simulink model "bus_as_currentsource_charging_discharging_battery_1"  (R2023a)
settings: Solver=VariableStepAuto  StartTime=0.0  StopTime=0.01  RelTol=1e-3
libraries: spsParallelRLCBranchLib x72, spsCurrentMeasurementLib x27, spsVoltageMeasurementLib x27, spspowerguiLib x25, spsControlledVoltageSourceLib x24, spsVariableResistorLib x24, spsSeriesRLCBranchLib x6, spsMosfetLib x2, sdolib x1, spsControlledCurrentSourceLib x1, spsGroundLib x1
(part 3 of 4)

== system bus_as_currentsource_charging_discharging_battery_1/Subsystem24 ==
  Clock : Clock
  Controlled Voltage Source : spsControlledVoltageSourceLib/Controlled Voltage Source  Initialize=on  Source_Type=DC  Amplitude=0  Phase=0  Frequency=0  Measurements=None
  Current Measurement : spsCurrentMeasurementLib/Current Measurement  PhasorSimulation=off  OutputType=Complex  PSBequivalent=0
  Delay : Delay  DelayLength=1  InitialCondition=0
  Delay1 : Delay  DelayLength=1  InitialCondition=0
  From1 : From
  From3 : From
  Goto1 : Goto
  Integrator : Integrator
  MATLAB Function : MATLAB Function  TreatAsAtomicUnit=on
  MATLAB Function1 : MATLAB Function  TreatAsAtomicUnit=on
  MATLAB Function2 : MATLAB Function  TreatAsAtomicUnit=on
  Parallel RLC Branch : spsParallelRLCBranchLib/Parallel RLC Branch  LConnTagsString=a  RConnTagsString=__new0  BranchType=RC  Resistance=15.5e-3  Inductance=1e-3  SetiL0=off  InitialCurrent=0  Capacitance=1028.7  Setx0=off  InitialVoltage=0  Measurements=None
  Parallel RLC Branch1 : spsParallelRLCBranchLib/Parallel RLC Branch  LConnTagsString=a  RConnTagsString=__new0  BranchType=RC  Resistance=18.3e-3  Inductance=1e-3  SetiL0=off  InitialCurrent=0  Capacitance=5756.6  Setx0=off  InitialVoltage=0  Measurements=None
  Parallel RLC Branch2 : spsParallelRLCBranchLib/Parallel RLC Branch  LConnTagsString=a  RConnTagsString=__new0  BranchType=R  Resistance=1e9  Inductance=1e-3  SetiL0=off  InitialCurrent=0  Capacitance=5756.6  Setx0=off  InitialVoltage=0  Measurements=None
  Scope2 : Scope
  Scope3 : Scope
  Scope4 : Scope
  Variable Resistor : spsVariableResistorLib/Variable Resistor  Rabsmin=1e-3
      settings: LibrarySourceBlock=sps_lib/Passives/Variable Resistor
  Voltage Measurement1 : spsVoltageMeasurementLib/Voltage Measurement  PhasorSimulation=off  OutputType=Complex  PSBequivalent=0
  XY Graph : Record  FileSettingsInternal="{\"entries\":[{\"content\":{\"excelSettings\":{\"content\":{},\"type\":\"Streamout.ExcelSettings\"}},\"type\":\"Streamout.FileSettingStorage\",\"uuid\":\"c5b1bd46-5ad2-463b-b602-37259b8cdc8f\"}],\"packageUris\":[\"http://schema.mathworks.com/mf0/streamout_blocks/R2020a\"],\"version\":\"1.0\"}"  Layout=[1 1]  SignalsInternal="{\"entries\":[{\"content\":{\"signals\":[{\"content\":{\"blockPath\":[\"bus_as_currentsource_charging_discharging_battery_1/Subsystem24/XY Graph\"],\"dimensions\":[1],\"domain\":\"bus_as_currentsource_charging_discharging_battery_1/Subsystem24/XY Graph\",\"lineColor\":\"#64d413\",\"port\":1,\"sid\":[\"\"],\"signalID\":331,\"signalName\":\"MATLAB Function2\"},\"type\":\"RecordBlkView.Signal\",\"uuid\":\"53831fb7-9f58-4ff5-bfff-82d8b3aa7aac\"},{\"content\":{\"blockPath\":[\"bus_as_currentsource_charging_discharging_battery_1/Subsystem24/XY Graph\"],\"dimensions\":[1],\"domain\":\"bus_as_currentsource_charging_discharging_battery_1/Subsystem24/XY Graph\",\"lineColor\":\"#ff13a6\",\"port\":2,\"sid\":[\"\"],\"signalID\":335,\"signalName\":\"Voltage Measurement1\"},\"type\":\"RecordBlkView.Signal\",\"uuid\":\"f3f18b01-4fe8-49fc-91c3-b068602f11c8\"}]},\"type\":\"RecordBlkView.InputSignals\",\"uuid\":\"28f569b0-f03a-459d-a4e3-dabbf623ccbc\"}],\"packageUris\":[\"http://schema.mathworks.com/mf0/streamout_blocks/R2020a\"],\"version\":\"1.0\"}"  VisualizationBindings="{\"xyplotplugin\":{\"info\":[{\"series\":[],\"subplotID\":1}]}}"  CompatibilityTag=XY
  powergui1 : spspowerguiLib/powergui  Priority=1  SimulationMode=Discrete  SampleTime=2e-7  frequency=60  Iterations=50  frequencyindice=0  Pbase=100e6  ErrMax=1e-4  UnitsV=kV  UnitsW=MW  buscounter=0  FunctionMessages=off  echomessages=off  EnableUseOfTLC=off  CurrentSourceSwitches=off  DisableSnubberDevices=off  DisableRonSwitches=off  DisableVfSwitches=off  DisplayEquations=off  AutomaticDiscreteSolvers=off  SolverType=Tustin/Backward Euler (TBE)  Interpol=off  ExternalGateDelay=off  methode=off  Ts=100  x0status=blocks  SPID=on  SwTol=0  HookPort=off  NonlinearTolerance=1e-4  nMaxIteration=100  ContinueOnMaxIteration=off  RestoreLinks=warning  ResistiveCurrentMeasurement=off  Frange=[0:2:500]  Ylog=off  Xlog=on  ShowGrid=off  save=off  variable=ZData  structure=0  ZoomFFT=off  StartTime=0.0  cycles=1  DisplayStyle=1  fundamental=60  FreqAxis=off  MaxFrequency=1000  frequencyindicesteady=1  RmsSteady=1  display=off
  + : PMIOPort  Side=Right
  - : PMIOPort  Port=2  Side=Left
  wires:
  Current Measurement/1 -> Goto1/1
  From3/1 -> Scope3/1
  Voltage Measurement1/1 -> XY Graph/2, Scope2/1
  MATLAB Function2/1(SOC) -> Delay/1, XY Graph/1, Scope4/1
  From1/1 -> Integrator/1
  MATLAB Function/1(y) -> Controlled Voltage Source/1
  MATLAB Function1/1(y) -> Variable Resistor/1
  Integrator/1 -> MATLAB Function2/1(u), MATLAB Function/1(u)
  Clock/1 -> MATLAB Function2/2(time), MATLAB Function/2(time)
  MATLAB Function/2(SOC) -> Delay1/1, MATLAB Function1/1(SOC)
  Delay/1 -> MATLAB Function2/3(SOC1)
  Delay1/1 -> MATLAB Function/3(SOC1)
  connections:
  Variable Resistor/RConn1 -- Parallel RLC Branch/LConn1
  Parallel RLC Branch1/RConn1 -- Parallel RLC Branch2/LConn1 -- +/RConn1 -- Voltage Measurement1/LConn1
  Voltage Measurement1/LConn2 -- Parallel RLC Branch2/RConn1 -- -/RConn1 -- Current Measurement/LConn1
  Controlled Voltage Source/RConn1 -- Variable Resistor/LConn1
  Current Measurement/RConn1 -- Controlled Voltage Source/LConn1
  Parallel RLC Branch/RConn1 -- Parallel RLC Branch1/LConn1

== system bus_as_currentsource_charging_discharging_battery_1/Subsystem3 ==
  Clock : Clock
  Controlled Voltage Source : spsControlledVoltageSourceLib/Controlled Voltage Source  Initialize=on  Source_Type=DC  Amplitude=0  Phase=0  Frequency=0  Measurements=None
  Current Measurement : spsCurrentMeasurementLib/Current Measurement  PhasorSimulation=off  OutputType=Complex  PSBequivalent=0
  Delay : Delay  DelayLength=1  InitialCondition=0
  Delay1 : Delay  DelayLength=1  InitialCondition=0
  From1 : From
  From3 : From
  Goto1 : Goto
  Integrator : Integrator
  MATLAB Function : MATLAB Function  TreatAsAtomicUnit=on
  MATLAB Function1 : MATLAB Function  TreatAsAtomicUnit=on
  MATLAB Function2 : MATLAB Function  TreatAsAtomicUnit=on
  Parallel RLC Branch : spsParallelRLCBranchLib/Parallel RLC Branch  LConnTagsString=a  RConnTagsString=__new0  BranchType=RC  Resistance=15.5e-3  Inductance=1e-3  SetiL0=off  InitialCurrent=0  Capacitance=1028.7  Setx0=off  InitialVoltage=0  Measurements=None
  Parallel RLC Branch1 : spsParallelRLCBranchLib/Parallel RLC Branch  LConnTagsString=a  RConnTagsString=__new0  BranchType=RC  Resistance=18.3e-3  Inductance=1e-3  SetiL0=off  InitialCurrent=0  Capacitance=5756.6  Setx0=off  InitialVoltage=0  Measurements=None
  Parallel RLC Branch2 : spsParallelRLCBranchLib/Parallel RLC Branch  LConnTagsString=a  RConnTagsString=__new0  BranchType=R  Resistance=1e9  Inductance=1e-3  SetiL0=off  InitialCurrent=0  Capacitance=5756.6  Setx0=off  InitialVoltage=0  Measurements=None
  Scope2 : Scope
  Scope3 : Scope
  Scope4 : Scope
  Variable Resistor : spsVariableResistorLib/Variable Resistor  Rabsmin=1e-3
      settings: LibrarySourceBlock=sps_lib/Passives/Variable Resistor
  Voltage Measurement1 : spsVoltageMeasurementLib/Voltage Measurement  PhasorSimulation=off  OutputType=Complex  PSBequivalent=0
  XY Graph : Record  FileSettingsInternal="{\"entries\":[{\"content\":{\"excelSettings\":{\"content\":{},\"type\":\"Streamout.ExcelSettings\"}},\"type\":\"Streamout.FileSettingStorage\",\"uuid\":\"9fe8c6ed-05dc-4d19-b685-e3030e54f32f\"}],\"packageUris\":[\"http://schema.mathworks.com/mf0/streamout_blocks/R2020a\"],\"version\":\"1.0\"}"  Layout=[1 1]  SignalsInternal="{\"entries\":[{\"content\":{\"signals\":[{\"content\":{\"blockPath\":[\"bus_as_currentsource_charging_discharging_battery_1/Subsystem3/XY Graph\"],\"dimensions\":[1],\"domain\":\"bus_as_currentsource_charging_discharging_battery_1/Subsystem3/XY Graph\",\"lineColor\":\"#fe330a\",\"port\":1,\"sid\":[\"\"],\"signalID\":339,\"signalName\":\"MATLAB Function2\"},\"type\":\"RecordBlkView.Signal\",\"uuid\":\"912f05b7-b733-407e-aac2-3b7bfc50d8b2\"},{\"content\":{\"blockPath\":[\"bus_as_currentsource_charging_discharging_battery_1/Subsystem3/XY Graph\"],\"dimensions\":[1],\"domain\":\"bus_as_currentsource_charging_discharging_battery_1/Subsystem3/XY Graph\",\"lineColor\":\"#22b573\",\"port\":2,\"sid\":[\"\"],\"signalID\":343,\"signalName\":\"Voltage Measurement1\"},\"type\":\"RecordBlkView.Signal\",\"uuid\":\"e02dbb8f-4be5-48ce-9df2-7af550d7c456\"}]},\"type\":\"RecordBlkView.InputSignals\",\"uuid\":\"dbab4033-9018-4bfc-9324-a303006a4a31\"}],\"packageUris\":[\"http://schema.mathworks.com/mf0/streamout_blocks/R2020a\"],\"version\":\"1.0\"}"  VisualizationBindings="{\"xyplotplugin\":{\"info\":[{\"series\":[],\"subplotID\":1}]}}"  CompatibilityTag=XY
  powergui1 : spspowerguiLib/powergui  Priority=1  SimulationMode=Discrete  SampleTime=2e-7  frequency=60  Iterations=50  frequencyindice=0  Pbase=100e6  ErrMax=1e-4  UnitsV=kV  UnitsW=MW  buscounter=0  FunctionMessages=off  echomessages=off  EnableUseOfTLC=off  CurrentSourceSwitches=off  DisableSnubberDevices=off  DisableRonSwitches=off  DisableVfSwitches=off  DisplayEquations=off  AutomaticDiscreteSolvers=off  SolverType=Tustin/Backward Euler (TBE)  Interpol=off  ExternalGateDelay=off  methode=off  Ts=100  x0status=blocks  SPID=on  SwTol=0  HookPort=off  NonlinearTolerance=1e-4  nMaxIteration=100  ContinueOnMaxIteration=off  RestoreLinks=warning  ResistiveCurrentMeasurement=off  Frange=[0:2:500]  Ylog=off  Xlog=on  ShowGrid=off  save=off  variable=ZData  structure=0  ZoomFFT=off  StartTime=0.0  cycles=1  DisplayStyle=1  fundamental=60  FreqAxis=off  MaxFrequency=1000  frequencyindicesteady=1  RmsSteady=1  display=off
  + : PMIOPort  Side=Right
  - : PMIOPort  Port=2  Side=Left
  wires:
  Current Measurement/1 -> Goto1/1
  From3/1 -> Scope3/1
  Voltage Measurement1/1 -> XY Graph/2, Scope2/1
  MATLAB Function2/1(SOC) -> Delay/1, XY Graph/1, Scope4/1
  From1/1 -> Integrator/1
  MATLAB Function/1(y) -> Controlled Voltage Source/1
  MATLAB Function1/1(y) -> Variable Resistor/1
  Integrator/1 -> MATLAB Function2/1(u), MATLAB Function/1(u)
  Clock/1 -> MATLAB Function2/2(time), MATLAB Function/2(time)
  MATLAB Function/2(SOC) -> Delay1/1, MATLAB Function1/1(SOC)
  Delay/1 -> MATLAB Function2/3(SOC1)
  Delay1/1 -> MATLAB Function/3(SOC1)
  connections:
  Variable Resistor/RConn1 -- Parallel RLC Branch/LConn1
  Parallel RLC Branch1/RConn1 -- Parallel RLC Branch2/LConn1 -- +/RConn1 -- Voltage Measurement1/LConn1
  Voltage Measurement1/LConn2 -- Parallel RLC Branch2/RConn1 -- -/RConn1 -- Current Measurement/LConn1
  Controlled Voltage Source/RConn1 -- Variable Resistor/LConn1
  Current Measurement/RConn1 -- Controlled Voltage Source/LConn1
  Parallel RLC Branch/RConn1 -- Parallel RLC Branch1/LConn1

== system bus_as_currentsource_charging_discharging_battery_1/Subsystem4 ==
  Clock : Clock
  Controlled Voltage Source : spsControlledVoltageSourceLib/Controlled Voltage Source  Initialize=on  Source_Type=DC  Amplitude=0  Phase=0  Frequency=0  Measurements=None
  Current Measurement : spsCurrentMeasurementLib/Current Measurement  PhasorSimulation=off  OutputType=Complex  PSBequivalent=0
  Delay : Delay  DelayLength=1  InitialCondition=0
  Delay1 : Delay  DelayLength=1  InitialCondition=0
  From1 : From
  From3 : From
  Goto1 : Goto
  Integrator : Integrator
  MATLAB Function : MATLAB Function  TreatAsAtomicUnit=on
  MATLAB Function1 : MATLAB Function  TreatAsAtomicUnit=on
  MATLAB Function2 : MATLAB Function  TreatAsAtomicUnit=on
  Parallel RLC Branch : spsParallelRLCBranchLib/Parallel RLC Branch  LConnTagsString=a  RConnTagsString=__new0  BranchType=RC  Resistance=15.5e-3  Inductance=1e-3  SetiL0=off  InitialCurrent=0  Capacitance=1028.7  Setx0=off  InitialVoltage=0  Measurements=None
  Parallel RLC Branch1 : spsParallelRLCBranchLib/Parallel RLC Branch  LConnTagsString=a  RConnTagsString=__new0  BranchType=RC  Resistance=18.3e-3  Inductance=1e-3  SetiL0=off  InitialCurrent=0  Capacitance=5756.6  Setx0=off  InitialVoltage=0  Measurements=None
  Parallel RLC Branch2 : spsParallelRLCBranchLib/Parallel RLC Branch  LConnTagsString=a  RConnTagsString=__new0  BranchType=R  Resistance=1e9  Inductance=1e-3  SetiL0=off  InitialCurrent=0  Capacitance=5756.6  Setx0=off  InitialVoltage=0  Measurements=None
  Scope2 : Scope
  Scope3 : Scope
  Scope4 : Scope
  Variable Resistor : spsVariableResistorLib/Variable Resistor  Rabsmin=1e-3
      settings: LibrarySourceBlock=sps_lib/Passives/Variable Resistor
  Voltage Measurement1 : spsVoltageMeasurementLib/Voltage Measurement  PhasorSimulation=off  OutputType=Complex  PSBequivalent=0
  XY Graph : Record  FileSettingsInternal="{\"entries\":[{\"content\":{\"excelSettings\":{\"content\":{},\"type\":\"Streamout.ExcelSettings\"}},\"type\":\"Streamout.FileSettingStorage\",\"uuid\":\"1c362e8b-adeb-4d87-81e4-7a7303bf4885\"}],\"packageUris\":[\"http://schema.mathworks.com/mf0/streamout_blocks/R2020a\"],\"version\":\"1.0\"}"  Layout=[1 1]  SignalsInternal="{\"entries\":[{\"content\":{\"signals\":[{\"content\":{\"blockPath\":[\"bus_as_currentsource_charging_discharging_battery_1/Subsystem4/XY Graph\"],\"dimensions\":[1],\"domain\":\"bus_as_currentsource_charging_discharging_battery_1/Subsystem4/XY Graph\",\"lineColor\":\"#0072bd\",\"port\":1,\"sid\":[\"\"],\"signalID\":347,\"signalName\":\"MATLAB Function2\"},\"type\":\"RecordBlkView.Signal\",\"uuid\":\"1b0b1bf4-064d-41fa-ba28-799bd76e9fc5\"},{\"content\":{\"blockPath\":[\"bus_as_currentsource_charging_discharging_battery_1/Subsystem4/XY Graph\"],\"dimensions\":[1],\"domain\":\"bus_as_currentsource_charging_discharging_battery_1/Subsystem4/XY Graph\",\"lineColor\":\"#d95319\",\"port\":2,\"sid\":[\"\"],\"signalID\":351,\"signalName\":\"Voltage Measurement1\"},\"type\":\"RecordBlkView.Signal\",\"uuid\":\"9899d34a-06e2-493a-970c-d9d2a010336a\"}]},\"type\":\"RecordBlkView.InputSignals\",\"uuid\":\"fc9c43f0-bf4a-40a4-8408-13b66da52628\"}],\"packageUris\":[\"http://schema.mathworks.com/mf0/streamout_blocks/R2020a\"],\"version\":\"1.0\"}"  VisualizationBindings="{\"xyplotplugin\":{\"info\":[{\"series\":[],\"subplotID\":1}]}}"  CompatibilityTag=XY
  powergui1 : spspowerguiLib/powergui  Priority=1  SimulationMode=Discrete  SampleTime=2e-7  frequency=60  Iterations=50  frequencyindice=0  Pbase=100e6  ErrMax=1e-4  UnitsV=kV  UnitsW=MW  buscounter=0  FunctionMessages=off  echomessages=off  EnableUseOfTLC=off  CurrentSourceSwitches=off  DisableSnubberDevices=off  DisableRonSwitches=off  DisableVfSwitches=off  DisplayEquations=off  AutomaticDiscreteSolvers=off  SolverType=Tustin/Backward Euler (TBE)  Interpol=off  ExternalGateDelay=off  methode=off  Ts=100  x0status=blocks  SPID=on  SwTol=0  HookPort=off  NonlinearTolerance=1e-4  nMaxIteration=100  ContinueOnMaxIteration=off  RestoreLinks=warning  ResistiveCurrentMeasurement=off  Frange=[0:2:500]  Ylog=off  Xlog=on  ShowGrid=off  save=off  variable=ZData  structure=0  ZoomFFT=off  StartTime=0.0  cycles=1  DisplayStyle=1  fundamental=60  FreqAxis=off  MaxFrequency=1000  frequencyindicesteady=1  RmsSteady=1  display=off
  + : PMIOPort  Side=Right
  - : PMIOPort  Port=2  Side=Left
  wires:
  Current Measurement/1 -> Goto1/1
  From3/1 -> Scope3/1
  Voltage Measurement1/1 -> XY Graph/2, Scope2/1
  MATLAB Function2/1(SOC) -> Delay/1, XY Graph/1, Scope4/1
  From1/1 -> Integrator/1
  MATLAB Function/1(y) -> Controlled Voltage Source/1
  MATLAB Function1/1(y) -> Variable Resistor/1
  Integrator/1 -> MATLAB Function2/1(u), MATLAB Function/1(u)
  Clock/1 -> MATLAB Function2/2(time), MATLAB Function/2(time)
  MATLAB Function/2(SOC) -> Delay1/1, MATLAB Function1/1(SOC)
  Delay/1 -> MATLAB Function2/3(SOC1)
  Delay1/1 -> MATLAB Function/3(SOC1)
  connections:
  Variable Resistor/RConn1 -- Parallel RLC Branch/LConn1
  Parallel RLC Branch1/RConn1 -- Parallel RLC Branch2/LConn1 -- +/RConn1 -- Voltage Measurement1/LConn1
  Voltage Measurement1/LConn2 -- Parallel RLC Branch2/RConn1 -- -/RConn1 -- Current Measurement/LConn1
  Controlled Voltage Source/RConn1 -- Variable Resistor/LConn1
  Current Measurement/RConn1 -- Controlled Voltage Source/LConn1
  Parallel RLC Branch/RConn1 -- Parallel RLC Branch1/LConn1

== system bus_as_currentsource_charging_discharging_battery_1/Subsystem5 ==
  Clock : Clock
  Controlled Voltage Source : spsControlledVoltageSourceLib/Controlled Voltage Source  Initialize=on  Source_Type=DC  Amplitude=0  Phase=0  Frequency=0  Measurements=None
  Current Measurement : spsCurrentMeasurementLib/Current Measurement  PhasorSimulation=off  OutputType=Complex  PSBequivalent=0
  Delay : Delay  DelayLength=1  InitialCondition=0
  Delay1 : Delay  DelayLength=1  InitialCondition=0
  From1 : From
  From3 : From
  Goto1 : Goto
  Integrator : Integrator
  MATLAB Function : MATLAB Function  TreatAsAtomicUnit=on
  MATLAB Function1 : MATLAB Function  TreatAsAtomicUnit=on
  MATLAB Function2 : MATLAB Function  TreatAsAtomicUnit=on
  Parallel RLC Branch : spsParallelRLCBranchLib/Parallel RLC Branch  LConnTagsString=a  RConnTagsString=__new0  BranchType=RC  Resistance=15.5e-3  Inductance=1e-3  SetiL0=off  InitialCurrent=0  Capacitance=1028.7  Setx0=off  InitialVoltage=0  Measurements=None
  Parallel RLC Branch1 : spsParallelRLCBranchLib/Parallel RLC Branch  LConnTagsString=a  RConnTagsString=__new0  BranchType=RC  Resistance=18.3e-3  Inductance=1e-3  SetiL0=off  InitialCurrent=0  Capacitance=5756.6  Setx0=off  InitialVoltage=0  Measurements=None
  Parallel RLC Branch2 : spsParallelRLCBranchLib/Parallel RLC Branch  LConnTagsString=a  RConnTagsString=__new0  BranchType=R  Resistance=1e9  Inductance=1e-3  SetiL0=off  InitialCurrent=0  Capacitance=5756.6  Setx0=off  InitialVoltage=0  Measurements=None
  Scope2 : Scope
  Scope3 : Scope
  Scope4 : Scope
  Variable Resistor : spsVariableResistorLib/Variable Resistor  Rabsmin=1e-3
      settings: LibrarySourceBlock=sps_lib/Passives/Variable Resistor
  Voltage Measurement1 : spsVoltageMeasurementLib/Voltage Measurement  PhasorSimulation=off  OutputType=Complex  PSBequivalent=0
  XY Graph : Record  FileSettingsInternal="{\"entries\":[{\"content\":{\"excelSettings\":{\"content\":{},\"type\":\"Streamout.ExcelSettings\"}},\"type\":\"Streamout.FileSettingStorage\",\"uuid\":\"0b3349e5-616a-4d30-ae5e-362adeb1e89f\"}],\"packageUris\":[\"http://schema.mathworks.com/mf0/streamout_blocks/R2020a\"],\"version\":\"1.0\"}"  Layout=[1 1]  SignalsInternal="{\"entries\":[{\"content\":{\"signals\":[{\"content\":{\"blockPath\":[\"bus_as_currentsource_charging_discharging_battery_1/Subsystem5/XY Graph\"],\"dimensions\":[1],\"domain\":\"bus_as_currentsource_charging_discharging_battery_1/Subsystem5/XY Graph\",\"lineColor\":\"#edb120\",\"port\":1,\"sid\":[\"\"],\"signalID\":355,\"signalName\":\"MATLAB Function2\"},\"type\":\"RecordBlkView.Signal\",\"uuid\":\"240c64b1-8fb4-4963-bedd-3d1886f7e516\"},{\"content\":{\"blockPath\":[\"bus_as_currentsource_charging_discharging_battery_1/Subsystem5/XY Graph\"],\"dimensions\":[1],\"domain\":\"bus_as_currentsource_charging_discharging_battery_1/Subsystem5/XY Graph\",\"lineColor\":\"#7e2f8e\",\"port\":2,\"sid\":[\"\"],\"signalID\":359,\"signalName\":\"Voltage Measurement1\"},\"type\":\"RecordBlkView.Signal\",\"uuid\":\"f1fef227-3787-4a48-b9c3-82269f12e824\"}]},\"type\":\"RecordBlkView.InputSignals\",\"uuid\":\"7cbcde80-bcd4-4066-b33f-54356b233c32\"}],\"packageUris\":[\"http://schema.mathworks.com/mf0/streamout_blocks/R2020a\"],\"version\":\"1.0\"}"  VisualizationBindings="{\"xyplotplugin\":{\"info\":[{\"series\":[],\"subplotID\":1}]}}"  CompatibilityTag=XY
  powergui1 : spspowerguiLib/powergui  Priority=1  SimulationMode=Discrete  SampleTime=2e-7  frequency=60  Iterations=50  frequencyindice=0  Pbase=100e6  ErrMax=1e-4  UnitsV=kV  UnitsW=MW  buscounter=0  FunctionMessages=off  echomessages=off  EnableUseOfTLC=off  CurrentSourceSwitches=off  DisableSnubberDevices=off  DisableRonSwitches=off  DisableVfSwitches=off  DisplayEquations=off  AutomaticDiscreteSolvers=off  SolverType=Tustin/Backward Euler (TBE)  Interpol=off  ExternalGateDelay=off  methode=off  Ts=100  x0status=blocks  SPID=on  SwTol=0  HookPort=off  NonlinearTolerance=1e-4  nMaxIteration=100  ContinueOnMaxIteration=off  RestoreLinks=warning  ResistiveCurrentMeasurement=off  Frange=[0:2:500]  Ylog=off  Xlog=on  ShowGrid=off  save=off  variable=ZData  structure=0  ZoomFFT=off  StartTime=0.0  cycles=1  DisplayStyle=1  fundamental=60  FreqAxis=off  MaxFrequency=1000  frequencyindicesteady=1  RmsSteady=1  display=off
  + : PMIOPort  Side=Right
  - : PMIOPort  Port=2  Side=Left
  wires:
  Current Measurement/1 -> Goto1/1
  From3/1 -> Scope3/1
  Voltage Measurement1/1 -> XY Graph/2, Scope2/1
  MATLAB Function2/1(SOC) -> Delay/1, XY Graph/1, Scope4/1
  From1/1 -> Integrator/1
  MATLAB Function/1(y) -> Controlled Voltage Source/1
  MATLAB Function1/1(y) -> Variable Resistor/1
  Integrator/1 -> MATLAB Function2/1(u), MATLAB Function/1(u)
  Clock/1 -> MATLAB Function2/2(time), MATLAB Function/2(time)
  MATLAB Function/2(SOC) -> Delay1/1, MATLAB Function1/1(SOC)
  Delay/1 -> MATLAB Function2/3(SOC1)
  Delay1/1 -> MATLAB Function/3(SOC1)
  connections:
  Variable Resistor/RConn1 -- Parallel RLC Branch/LConn1
  Parallel RLC Branch1/RConn1 -- Parallel RLC Branch2/LConn1 -- +/RConn1 -- Voltage Measurement1/LConn1
  Voltage Measurement1/LConn2 -- Parallel RLC Branch2/RConn1 -- -/RConn1 -- Current Measurement/LConn1
  Controlled Voltage Source/RConn1 -- Variable Resistor/LConn1
  Current Measurement/RConn1 -- Controlled Voltage Source/LConn1
  Parallel RLC Branch/RConn1 -- Parallel RLC Branch1/LConn1

== system bus_as_currentsource_charging_discharging_battery_1/Subsystem6 ==
  Clock : Clock
  Controlled Voltage Source : spsControlledVoltageSourceLib/Controlled Voltage Source  Initialize=on  Source_Type=DC  Amplitude=0  Phase=0  Frequency=0  Measurements=None
  Current Measurement : spsCurrentMeasurementLib/Current Measurement  PhasorSimulation=off  OutputType=Complex  PSBequivalent=0
  Delay : Delay  DelayLength=1  InitialCondition=0
  Delay1 : Delay  DelayLength=1  InitialCondition=0
  From1 : From
  From3 : From
  Goto1 : Goto
  Integrator : Integrator
  MATLAB Function : MATLAB Function  TreatAsAtomicUnit=on
  MATLAB Function1 : MATLAB Function  TreatAsAtomicUnit=on
  MATLAB Function2 : MATLAB Function  TreatAsAtomicUnit=on
  Parallel RLC Branch : spsParallelRLCBranchLib/Parallel RLC Branch  LConnTagsString=a  RConnTagsString=__new0  BranchType=RC  Resistance=15.5e-3  Inductance=1e-3  SetiL0=off  InitialCurrent=0  Capacitance=1028.7  Setx0=off  InitialVoltage=0  Measurements=None
  Parallel RLC Branch1 : spsParallelRLCBranchLib/Parallel RLC Branch  LConnTagsString=a  RConnTagsString=__new0  BranchType=RC  Resistance=18.3e-3  Inductance=1e-3  SetiL0=off  InitialCurrent=0  Capacitance=5756.6  Setx0=off  InitialVoltage=0  Measurements=None
  Parallel RLC Branch2 : spsParallelRLCBranchLib/Parallel RLC Branch  LConnTagsString=a  RConnTagsString=__new0  BranchType=R  Resistance=1e9  Inductance=1e-3  SetiL0=off  InitialCurrent=0  Capacitance=5756.6  Setx0=off  InitialVoltage=0  Measurements=None
  Scope2 : Scope
  Scope3 : Scope
  Scope4 : Scope
  Variable Resistor : spsVariableResistorLib/Variable Resistor  Rabsmin=1e-3
      settings: LibrarySourceBlock=sps_lib/Passives/Variable Resistor
  Voltage Measurement1 : spsVoltageMeasurementLib/Voltage Measurement  PhasorSimulation=off  OutputType=Complex  PSBequivalent=0
  XY Graph : Record  FileSettingsInternal="{\"entries\":[{\"content\":{\"excelSettings\":{\"content\":{},\"type\":\"Streamout.ExcelSettings\"}},\"type\":\"Streamout.FileSettingStorage\",\"uuid\":\"704fec78-3d60-48ee-ad59-a61ce2d31f0a\"}],\"packageUris\":[\"http://schema.mathworks.com/mf0/streamout_blocks/R2020a\"],\"version\":\"1.0\"}"  Layout=[1 1]  SignalsInternal="{\"entries\":[{\"content\":{\"signals\":[{\"content\":{\"blockPath\":[\"bus_as_currentsource_charging_discharging_battery_1/Subsystem6/XY Graph\"],\"dimensions\":[1],\"domain\":\"bus_as_currentsource_charging_discharging_battery_1/Subsystem6/XY Graph\",\"lineColor\":\"#77ac30\",\"port\":1,\"sid\":[\"\"],\"signalID\":363,\"signalName\":\"MATLAB Function2\"},\"type\":\"RecordBlkView.Signal\",\"uuid\":\"74a4a9b1-61a0-483e-844c-8e414649572f\"},{\"content\":{\"blockPath\":[\"bus_as_currentsource_charging_discharging_battery_1/Subsystem6/XY Graph\"],\"dimensions\":[1],\"domain\":\"bus_as_currentsource_charging_discharging_battery_1/Subsystem6/XY Graph\",\"lineColor\":\"#4dbeee\",\"port\":2,\"sid\":[\"\"],\"signalID\":367,\"signalName\":\"Voltage Measurement1\"},\"type\":\"RecordBlkView.Signal\",\"uuid\":\"19bc8c94-5366-4b4c-92f5-c2fba838555b\"}]},\"type\":\"RecordBlkView.InputSignals\",\"uuid\":\"7e0e1a44-64e9-42f4-be90-734e24720156\"}],\"packageUris\":[\"http://schema.mathworks.com/mf0/streamout_blocks/R2020a\"],\"version\":\"1.0\"}"  VisualizationBindings="{\"xyplotplugin\":{\"info\":[{\"series\":[],\"subplotID\":1}]}}"  CompatibilityTag=XY
  powergui1 : spspowerguiLib/powergui  Priority=1  SimulationMode=Discrete  SampleTime=2e-7  frequency=60  Iterations=50  frequencyindice=0  Pbase=100e6  ErrMax=1e-4  UnitsV=kV  UnitsW=MW  buscounter=0  FunctionMessages=off  echomessages=off  EnableUseOfTLC=off  CurrentSourceSwitches=off  DisableSnubberDevices=off  DisableRonSwitches=off  DisableVfSwitches=off  DisplayEquations=off  AutomaticDiscreteSolvers=off  SolverType=Tustin/Backward Euler (TBE)  Interpol=off  ExternalGateDelay=off  methode=off  Ts=100  x0status=blocks  SPID=on  SwTol=0  HookPort=off  NonlinearTolerance=1e-4  nMaxIteration=100  ContinueOnMaxIteration=off  RestoreLinks=warning  ResistiveCurrentMeasurement=off  Frange=[0:2:500]  Ylog=off  Xlog=on  ShowGrid=off  save=off  variable=ZData  structure=0  ZoomFFT=off  StartTime=0.0  cycles=1  DisplayStyle=1  fundamental=60  FreqAxis=off  MaxFrequency=1000  frequencyindicesteady=1  RmsSteady=1  display=off
  + : PMIOPort  Side=Right
  - : PMIOPort  Port=2  Side=Left
  wires:
  Current Measurement/1 -> Goto1/1
  From3/1 -> Scope3/1
  Voltage Measurement1/1 -> XY Graph/2, Scope2/1
  MATLAB Function2/1(SOC) -> Delay/1, XY Graph/1, Scope4/1
  From1/1 -> Integrator/1
  MATLAB Function/1(y) -> Controlled Voltage Source/1
  MATLAB Function1/1(y) -> Variable Resistor/1
  Integrator/1 -> MATLAB Function2/1(u), MATLAB Function/1(u)
  Clock/1 -> MATLAB Function2/2(time), MATLAB Function/2(time)
  MATLAB Function/2(SOC) -> Delay1/1, MATLAB Function1/1(SOC)
  Delay/1 -> MATLAB Function2/3(SOC1)
  Delay1/1 -> MATLAB Function/3(SOC1)
  connections:
  Variable Resistor/RConn1 -- Parallel RLC Branch/LConn1
  Parallel RLC Branch1/RConn1 -- Parallel RLC Branch2/LConn1 -- +/RConn1 -- Voltage Measurement1/LConn1
  Voltage Measurement1/LConn2 -- Parallel RLC Branch2/RConn1 -- -/RConn1 -- Current Measurement/LConn1
  Controlled Voltage Source/RConn1 -- Variable Resistor/LConn1
  Current Measurement/RConn1 -- Controlled Voltage Source/LConn1
  Parallel RLC Branch/RConn1 -- Parallel RLC Branch1/LConn1

== system bus_as_currentsource_charging_discharging_battery_1/Subsystem7 ==
  Clock : Clock
  Controlled Voltage Source : spsControlledVoltageSourceLib/Controlled Voltage Source  Initialize=on  Source_Type=DC  Amplitude=0  Phase=0  Frequency=0  Measurements=None
  Current Measurement : spsCurrentMeasurementLib/Current Measurement  PhasorSimulation=off  OutputType=Complex  PSBequivalent=0
  Delay : Delay  DelayLength=1  InitialCondition=0
  Delay1 : Delay  DelayLength=1  InitialCondition=0
  From1 : From
  From3 : From
  Goto1 : Goto
  Integrator : Integrator
  MATLAB Function : MATLAB Function  TreatAsAtomicUnit=on
  MATLAB Function1 : MATLAB Function  TreatAsAtomicUnit=on
  MATLAB Function2 : MATLAB Function  TreatAsAtomicUnit=on
  Parallel RLC Branch : spsParallelRLCBranchLib/Parallel RLC Branch  LConnTagsString=a  RConnTagsString=__new0  BranchType=RC  Resistance=15.5e-3  Inductance=1e-3  SetiL0=off  InitialCurrent=0  Capacitance=1028.7  Setx0=off  InitialVoltage=0  Measurements=None
  Parallel RLC Branch1 : spsParallelRLCBranchLib/Parallel RLC Branch  LConnTagsString=a  RConnTagsString=__new0  BranchType=RC  Resistance=18.3e-3  Inductance=1e-3  SetiL0=off  InitialCurrent=0  Capacitance=5756.6  Setx0=off  InitialVoltage=0  Measurements=None
  Parallel RLC Branch2 : spsParallelRLCBranchLib/Parallel RLC Branch  LConnTagsString=a  RConnTagsString=__new0  BranchType=R  Resistance=1e9  Inductance=1e-3  SetiL0=off  InitialCurrent=0  Capacitance=5756.6  Setx0=off  InitialVoltage=0  Measurements=None
  Scope2 : Scope
  Scope3 : Scope
  Scope4 : Scope
  Variable Resistor : spsVariableResistorLib/Variable Resistor  Rabsmin=1e-3
      settings: LibrarySourceBlock=sps_lib/Passives/Variable Resistor
  Voltage Measurement1 : spsVoltageMeasurementLib/Voltage Measurement  PhasorSimulation=off  OutputType=Complex  PSBequivalent=0
  XY Graph : Record  FileSettingsInternal="{\"entries\":[{\"content\":{\"excelSettings\":{\"content\":{},\"type\":\"Streamout.ExcelSettings\"}},\"type\":\"Streamout.FileSettingStorage\",\"uuid\":\"f70bcb4a-5097-4ac6-8080-f37201fbaf57\"}],\"packageUris\":[\"http://schema.mathworks.com/mf0/streamout_blocks/R2020a\"],\"version\":\"1.0\"}"  Layout=[1 1]  SignalsInternal="{\"entries\":[{\"content\":{\"signals\":[{\"content\":{\"blockPath\":[\"bus_as_currentsource_charging_discharging_battery_1/Subsystem7/XY Graph\"],\"dimensions\":[1],\"domain\":\"bus_as_currentsource_charging_discharging_battery_1/Subsystem7/XY Graph\",\"lineColor\":\"#a2142f\",\"port\":1,\"sid\":[\"\"],\"signalID\":371,\"signalName\":\"MATLAB Function2\"},\"type\":\"RecordBlkView.Signal\",\"uuid\":\"bdf11a01-3d24-4955-b5d2-15773a9da791\"},{\"content\":{\"blockPath\":[\"bus_as_currentsource_charging_discharging_battery_1/Subsystem7/XY Graph\"],\"dimensions\":[1],\"domain\":\"bus_as_currentsource_charging_discharging_battery_1/Subsystem7/XY Graph\",\"lineColor\":\"#139fff\",\"port\":2,\"sid\":[\"\"],\"signalID\":375,\"signalName\":\"Voltage Measurement1\"},\"type\":\"RecordBlkView.Signal\",\"uuid\":\"a1710896-1f52-47e5-af89-08dc694cce8f\"}]},\"type\":\"RecordBlkView.InputSignals\",\"uuid\":\"de44fd4f-8b2d-4411-85f2-d2e0afef5e41\"}],\"packageUris\":[\"http://schema.mathworks.com/mf0/streamout_blocks/R2020a\"],\"version\":\"1.0\"}"  VisualizationBindings="{\"xyplotplugin\":{\"info\":[{\"series\":[],\"subplotID\":1}]}}"  CompatibilityTag=XY
  powergui1 : spspowerguiLib/powergui  Priority=1  SimulationMode=Discrete  SampleTime=2e-7  frequency=60  Iterations=50  frequencyindice=0  Pbase=100e6  ErrMax=1e-4  UnitsV=kV  UnitsW=MW  buscounter=0  FunctionMessages=off  echomessages=off  EnableUseOfTLC=off  CurrentSourceSwitches=off  DisableSnubberDevices=off  DisableRonSwitches=off  DisableVfSwitches=off  DisplayEquations=off  AutomaticDiscreteSolvers=off  SolverType=Tustin/Backward Euler (TBE)  Interpol=off  ExternalGateDelay=off  methode=off  Ts=100  x0status=blocks  SPID=on  SwTol=0  HookPort=off  NonlinearTolerance=1e-4  nMaxIteration=100  ContinueOnMaxIteration=off  RestoreLinks=warning  ResistiveCurrentMeasurement=off  Frange=[0:2:500]  Ylog=off  Xlog=on  ShowGrid=off  save=off  variable=ZData  structure=0  ZoomFFT=off  StartTime=0.0  cycles=1  DisplayStyle=1  fundamental=60  FreqAxis=off  MaxFrequency=1000  frequencyindicesteady=1  RmsSteady=1  display=off
  + : PMIOPort  Side=Right
  - : PMIOPort  Port=2  Side=Left
  wires:
  Current Measurement/1 -> Goto1/1
  From3/1 -> Scope3/1
  Voltage Measurement1/1 -> XY Graph/2, Scope2/1
  MATLAB Function2/1(SOC) -> Delay/1, XY Graph/1, Scope4/1
  From1/1 -> Integrator/1
  MATLAB Function/1(y) -> Controlled Voltage Source/1
  MATLAB Function1/1(y) -> Variable Resistor/1
  Integrator/1 -> MATLAB Function2/1(u), MATLAB Function/1(u)
  Clock/1 -> MATLAB Function2/2(time), MATLAB Function/2(time)
  MATLAB Function/2(SOC) -> Delay1/1, MATLAB Function1/1(SOC)
  Delay/1 -> MATLAB Function2/3(SOC1)
  Delay1/1 -> MATLAB Function/3(SOC1)
  connections:
  Variable Resistor/RConn1 -- Parallel RLC Branch/LConn1
  Parallel RLC Branch1/RConn1 -- Parallel RLC Branch2/LConn1 -- +/RConn1 -- Voltage Measurement1/LConn1
  Voltage Measurement1/LConn2 -- Parallel RLC Branch2/RConn1 -- -/RConn1 -- Current Measurement/LConn1
  Controlled Voltage Source/RConn1 -- Variable Resistor/LConn1
  Current Measurement/RConn1 -- Controlled Voltage Source/LConn1
  Parallel RLC Branch/RConn1 -- Parallel RLC Branch1/LConn1

== system bus_as_currentsource_charging_discharging_battery_1/Subsystem8 ==
  Clock : Clock
  Controlled Voltage Source : spsControlledVoltageSourceLib/Controlled Voltage Source  Initialize=on  Source_Type=DC  Amplitude=0  Phase=0  Frequency=0  Measurements=None
  Current Measurement : spsCurrentMeasurementLib/Current Measurement  PhasorSimulation=off  OutputType=Complex  PSBequivalent=0
  Delay : Delay  DelayLength=1  InitialCondition=0
  Delay1 : Delay  DelayLength=1  InitialCondition=0
  From1 : From
  From3 : From
  Goto1 : Goto
  Integrator : Integrator
  MATLAB Function : MATLAB Function  TreatAsAtomicUnit=on
  MATLAB Function1 : MATLAB Function  TreatAsAtomicUnit=on
  MATLAB Function2 : MATLAB Function  TreatAsAtomicUnit=on
  Parallel RLC Branch : spsParallelRLCBranchLib/Parallel RLC Branch  LConnTagsString=a  RConnTagsString=__new0  BranchType=RC  Resistance=15.5e-3  Inductance=1e-3  SetiL0=off  InitialCurrent=0  Capacitance=1028.7  Setx0=off  InitialVoltage=0  Measurements=None
  Parallel RLC Branch1 : spsParallelRLCBranchLib/Parallel RLC Branch  LConnTagsString=a  RConnTagsString=__new0  BranchType=RC  Resistance=18.3e-3  Inductance=1e-3  SetiL0=off  InitialCurrent=0  Capacitance=5756.6  Setx0=off  InitialVoltage=0  Measurements=None
  Parallel RLC Branch2 : spsParallelRLCBranchLib/Parallel RLC Branch  LConnTagsString=a  RConnTagsString=__new0  BranchType=R  Resistance=1e9  Inductance=1e-3  SetiL0=off  InitialCurrent=0  Capacitance=5756.6  Setx0=off  InitialVoltage=0  Measurements=None
  Scope2 : Scope
  Scope3 : Scope
  Scope4 : Scope
  Variable Resistor : spsVariableResistorLib/Variable Resistor  Rabsmin=1e-3
      settings: LibrarySourceBlock=sps_lib/Passives/Variable Resistor
  Voltage Measurement1 : spsVoltageMeasurementLib/Voltage Measurement  PhasorSimulation=off  OutputType=Complex  PSBequivalent=0
  XY Graph : Record  FileSettingsInternal="{\"entries\":[{\"content\":{\"excelSettings\":{\"content\":{},\"type\":\"Streamout.ExcelSettings\"}},\"type\":\"Streamout.FileSettingStorage\",\"uuid\":\"bab5c315-22ef-4102-80e8-0f9efa6107b0\"}],\"packageUris\":[\"http://schema.mathworks.com/mf0/streamout_blocks/R2020a\"],\"version\":\"1.0\"}"  Layout=[1 1]  SignalsInternal="{\"entries\":[{\"content\":{\"signals\":[{\"content\":{\"blockPath\":[\"bus_as_currentsource_charging_discharging_battery_1/Subsystem8/XY Graph\"],\"dimensions\":[1],\"domain\":\"bus_as_currentsource_charging_discharging_battery_1/Subsystem8/XY Graph\",\"lineColor\":\"#ff6929\",\"port\":1,\"sid\":[\"\"],\"signalID\":379,\"signalName\":\"MATLAB Function2\"},\"type\":\"RecordBlkView.Signal\",\"uuid\":\"088d50c4-cbb9-4ed5-b52f-57afd3ef5803\"},{\"content\":{\"blockPath\":[\"bus_as_currentsource_charging_discharging_battery_1/Subsystem8/XY Graph\"],\"dimensions\":[1],\"domain\":\"bus_as_currentsource_charging_discharging_battery_1/Subsystem8/XY Graph\",\"lineColor\":\"#b746ff\",\"port\":2,\"sid\":[\"\"],\"signalID\":383,\"signalName\":\"Voltage Measurement1\"},\"type\":\"RecordBlkView.Signal\",\"uuid\":\"5c455657-d4c6-423b-abdc-c2ab39cdb0cf\"}]},\"type\":\"RecordBlkView.InputSignals\",\"uuid\":\"84d414da-df6a-4aab-8207-09f98a22eff4\"}],\"packageUris\":[\"http://schema.mathworks.com/mf0/streamout_blocks/R2020a\"],\"version\":\"1.0\"}"  VisualizationBindings="{\"xyplotplugin\":{\"info\":[{\"series\":[],\"subplotID\":1}]}}"  CompatibilityTag=XY
  powergui1 : spspowerguiLib/powergui  Priority=1  SimulationMode=Discrete  SampleTime=2e-7  frequency=60  Iterations=50  frequencyindice=0  Pbase=100e6  ErrMax=1e-4  UnitsV=kV  UnitsW=MW  buscounter=0  FunctionMessages=off  echomessages=off  EnableUseOfTLC=off  CurrentSourceSwitches=off  DisableSnubberDevices=off  DisableRonSwitches=off  DisableVfSwitches=off  DisplayEquations=off  AutomaticDiscreteSolvers=off  SolverType=Tustin/Backward Euler (TBE)  Interpol=off  ExternalGateDelay=off  methode=off  Ts=100  x0status=blocks  SPID=on  SwTol=0  HookPort=off  NonlinearTolerance=1e-4  nMaxIteration=100  ContinueOnMaxIteration=off  RestoreLinks=warning  ResistiveCurrentMeasurement=off  Frange=[0:2:500]  Ylog=off  Xlog=on  ShowGrid=off  save=off  variable=ZData  structure=0  ZoomFFT=off  StartTime=0.0  cycles=1  DisplayStyle=1  fundamental=60  FreqAxis=off  MaxFrequency=1000  frequencyindicesteady=1  RmsSteady=1  display=off
  + : PMIOPort  Side=Right
  - : PMIOPort  Port=2  Side=Left
  wires:
  Current Measurement/1 -> Goto1/1
  From3/1 -> Scope3/1
  Voltage Measurement1/1 -> XY Graph/2, Scope2/1
  MATLAB Function2/1(SOC) -> Delay/1, XY Graph/1, Scope4/1
  From1/1 -> Integrator/1
  MATLAB Function/1(y) -> Controlled Voltage Source/1
  MATLAB Function1/1(y) -> Variable Resistor/1
  Integrator/1 -> MATLAB Function2/1(u), MATLAB Function/1(u)
  Clock/1 -> MATLAB Function2/2(time), MATLAB Function/2(time)
  MATLAB Function/2(SOC) -> Delay1/1, MATLAB Function1/1(SOC)
  Delay/1 -> MATLAB Function2/3(SOC1)
  Delay1/1 -> MATLAB Function/3(SOC1)
  connections:
  Variable Resistor/RConn1 -- Parallel RLC Branch/LConn1
  Parallel RLC Branch1/RConn1 -- Parallel RLC Branch2/LConn1 -- +/RConn1 -- Voltage Measurement1/LConn1
  Voltage Measurement1/LConn2 -- Parallel RLC Branch2/RConn1 -- -/RConn1 -- Current Measurement/LConn1
  Controlled Voltage Source/RConn1 -- Variable Resistor/LConn1
  Current Measurement/RConn1 -- Controlled Voltage Source/LConn1
  Parallel RLC Branch/RConn1 -- Parallel RLC Branch1/LConn1

== system bus_as_currentsource_charging_discharging_battery_1/Subsystem9 ==
  Clock : Clock
  Controlled Voltage Source : spsControlledVoltageSourceLib/Controlled Voltage Source  Initialize=on  Source_Type=DC  Amplitude=0  Phase=0  Frequency=0  Measurements=None
  Current Measurement : spsCurrentMeasurementLib/Current Measurement  PhasorSimulation=off  OutputType=Complex  PSBequivalent=0
  Delay : Delay  DelayLength=1  InitialCondition=0
  Delay1 : Delay  DelayLength=1  InitialCondition=0
  From1 : From
  From3 : From
  Goto1 : Goto
  Integrator : Integrator
  MATLAB Function : MATLAB Function  TreatAsAtomicUnit=on
  MATLAB Function1 : MATLAB Function  TreatAsAtomicUnit=on
  MATLAB Function2 : MATLAB Function  TreatAsAtomicUnit=on
  Parallel RLC Branch : spsParallelRLCBranchLib/Parallel RLC Branch  LConnTagsString=a  RConnTagsString=__new0  BranchType=RC  Resistance=15.5e-3  Inductance=1e-3  SetiL0=off  InitialCurrent=0  Capacitance=1028.7  Setx0=off  InitialVoltage=0  Measurements=None
  Parallel RLC Branch1 : spsParallelRLCBranchLib/Parallel RLC Branch  LConnTagsString=a  RConnTagsString=__new0  BranchType=RC  Resistance=18.3e-3  Inductance=1e-3  SetiL0=off  InitialCurrent=0  Capacitance=5756.6  Setx0=off  InitialVoltage=0  Measurements=None
  Parallel RLC Branch2 : spsParallelRLCBranchLib/Parallel RLC Branch  LConnTagsString=a  RConnTagsString=__new0  BranchType=R  Resistance=1e9  Inductance=1e-3  SetiL0=off  InitialCurrent=0  Capacitance=5756.6  Setx0=off  InitialVoltage=0  Measurements=None
  Scope2 : Scope
  Scope3 : Scope
  Scope4 : Scope
  Variable Resistor : spsVariableResistorLib/Variable Resistor  Rabsmin=1e-3
      settings: LibrarySourceBlock=sps_lib/Passives/Variable Resistor
  Voltage Measurement1 : spsVoltageMeasurementLib/Voltage Measurement  PhasorSimulation=off  OutputType=Complex  PSBequivalent=0
  XY Graph : Record  FileSettingsInternal="{\"entries\":[{\"content\":{\"excelSettings\":{\"content\":{},\"type\":\"Streamout.ExcelSettings\"}},\"type\":\"Streamout.FileSettingStorage\",\"uuid\":\"94df0f40-82d0-4655-a62b-73149d8160f3\"}],\"packageUris\":[\"http://schema.mathworks.com/mf0/streamout_blocks/R2020a\"],\"version\":\"1.0\"}"  Layout=[1 1]  SignalsInternal="{\"entries\":[{\"content\":{\"signals\":[{\"content\":{\"blockPath\":[\"bus_as_currentsource_charging_discharging_battery_1/Subsystem9/XY Graph\"],\"dimensions\":[1],\"domain\":\"bus_as_currentsource_charging_discharging_battery_1/Subsystem9/XY Graph\",\"lineColor\":\"#64d413\",\"port\":1,\"sid\":[\"\"],\"signalID\":387,\"signalName\":\"MATLAB Function2\"},\"type\":\"RecordBlkView.Signal\",\"uuid\":\"31e55c6b-47cc-43c5-a51a-7fa00ea2c876\"},{\"content\":{\"blockPath\":[\"bus_as_currentsource_charging_discharging_battery_1/Subsystem9/XY Graph\"],\"dimensions\":[1],\"domain\":\"bus_as_currentsource_charging_discharging_battery_1/Subsystem9/XY Graph\",\"lineColor\":\"#ff13a6\",\"port\":2,\"sid\":[\"\"],\"signalID\":391,\"signalName\":\"Voltage Measurement1\"},\"type\":\"RecordBlkView.Signal\",\"uuid\":\"c7d0580b-78f8-4d87-a713-1abc7979e9ae\"}]},\"type\":\"RecordBlkView.InputSignals\",\"uuid\":\"790e1e39-6d20-477e-8b82-bbd46e17942e\"}],\"packageUris\":[\"http://schema.mathworks.com/mf0/streamout_blocks/R2020a\"],\"version\":\"1.0\"}"  VisualizationBindings="{\"xyplotplugin\":{\"info\":[{\"series\":[],\"subplotID\":1}]}}"  CompatibilityTag=XY
  powergui1 : spspowerguiLib/powergui  Priority=1  SimulationMode=Discrete  SampleTime=2e-7  frequency=60  Iterations=50  frequencyindice=0  Pbase=100e6  ErrMax=1e-4  UnitsV=kV  UnitsW=MW  buscounter=0  FunctionMessages=off  echomessages=off  EnableUseOfTLC=off  CurrentSourceSwitches=off  DisableSnubberDevices=off  DisableRonSwitches=off  DisableVfSwitches=off  DisplayEquations=off  AutomaticDiscreteSolvers=off  SolverType=Tustin/Backward Euler (TBE)  Interpol=off  ExternalGateDelay=off  methode=off  Ts=100  x0status=blocks  SPID=on  SwTol=0  HookPort=off  NonlinearTolerance=1e-4  nMaxIteration=100  ContinueOnMaxIteration=off  RestoreLinks=warning  ResistiveCurrentMeasurement=off  Frange=[0:2:500]  Ylog=off  Xlog=on  ShowGrid=off  save=off  variable=ZData  structure=0  ZoomFFT=off  StartTime=0.0  cycles=1  DisplayStyle=1  fundamental=60  FreqAxis=off  MaxFrequency=1000  frequencyindicesteady=1  RmsSteady=1  display=off
  + : PMIOPort  Side=Right
  - : PMIOPort  Port=2  Side=Left
  wires:
  Current Measurement/1 -> Goto1/1
  From3/1 -> Scope3/1
  Voltage Measurement1/1 -> XY Graph/2, Scope2/1
  MATLAB Function2/1(SOC) -> Delay/1, XY Graph/1, Scope4/1
  From1/1 -> Integrator/1
  MATLAB Function/1(y) -> Controlled Voltage Source/1
  MATLAB Function1/1(y) -> Variable Resistor/1
  Integrator/1 -> MATLAB Function2/1(u), MATLAB Function/1(u)
  Clock/1 -> MATLAB Function2/2(time), MATLAB Function/2(time)
  MATLAB Function/2(SOC) -> Delay1/1, MATLAB Function1/1(SOC)
  Delay/1 -> MATLAB Function2/3(SOC1)
  Delay1/1 -> MATLAB Function/3(SOC1)
  connections:
  Variable Resistor/RConn1 -- Parallel RLC Branch/LConn1
  Parallel RLC Branch1/RConn1 -- Parallel RLC Branch2/LConn1 -- +/RConn1 -- Voltage Measurement1/LConn1
  Voltage Measurement1/LConn2 -- Parallel RLC Branch2/RConn1 -- -/RConn1 -- Current Measurement/LConn1
  Controlled Voltage Source/RConn1 -- Variable Resistor/LConn1
  Current Measurement/RConn1 -- Controlled Voltage Source/LConn1
  Parallel RLC Branch/RConn1 -- Parallel RLC Branch1/LConn1

== matlab function bus_as_currentsource_charging_discharging_battery_1/Subsystem1/MATLAB Function ==
  data: u input; y output; time input; SOC output; SOC1 input
function [y,SOC]= fcn(u,time,SOC1)
if time <0.006
    SOC= 60 + 60*u/7920;
else
    SOC=SOC1-SOC1*u/7920;
end
y = 5.56e-5.*SOC.^2+0.001788.*SOC+3.491;

== matlab function bus_as_currentsource_charging_discharging_battery_1/Subsystem4/MATLAB Function2 ==
  data: u input; SOC output; time input; SOC1 input
function SOC= fcn(u,time,SOC1)
if time <0.006
    SOC= 60 + 60*u/7920;
else
    SOC=SOC1-SOC1*u/7920;
end

== matlab function bus_as_currentsource_charging_discharging_battery_1/Subsystem5/MATLAB Function ==
  data: u input; y output; time input; SOC output; SOC1 input
function [y,SOC]= fcn(u,time,SOC1)
if time <0.006
    SOC= 60 + 60*u/7920;
else
    SOC=SOC1-SOC1*u/7920;
end
y = 5.56e-5.*SOC.^2+0.001788.*SOC+3.491;

== matlab function bus_as_currentsource_charging_discharging_battery_1/Subsystem5/MATLAB Function1 ==
  data: SOC input; y output
function y = fcn(SOC)
p1=2.229e-9;
p2=-5.378e-7;
p3=4.791e-5;
p4=-0.001908;
p5=0.08808;
y=p1*SOC^4+p2*SOC^3+p3*SOC^2+p4*SOC+p5;

== matlab function bus_as_currentsource_charging_discharging_battery_1/Subsystem5/MATLAB Function2 ==
  data: u input; SOC output; time input; SOC1 input
function SOC= fcn(u,time,SOC1)
if time <0.006
    SOC= 60 + 60*u/7920;
else
    SOC=SOC1-SOC1*u/7920;
end

== matlab function bus_as_currentsource_charging_discharging_battery_1/Subsystem6/MATLAB Function ==
  data: u input; y output; time input; SOC output; SOC1 input
function [y,SOC]= fcn(u,time,SOC1)
if time <0.006
    SOC= 60 + 60*u/7920;
else
    SOC=SOC1-SOC1*u/7920;
end
y = 5.56e-5.*SOC.^2+0.001788.*SOC+3.491;

== matlab function bus_as_currentsource_charging_discharging_battery_1/Subsystem6/MATLAB Function1 ==
  data: SOC input; y output
function y = fcn(SOC)
p1=2.229e-9;
p2=-5.378e-7;
p3=4.791e-5;
p4=-0.001908;
p5=0.08808;
y=p1*SOC^4+p2*SOC^3+p3*SOC^2+p4*SOC+p5;

== matlab function bus_as_currentsource_charging_discharging_battery_1/Subsystem6/MATLAB Function2 ==
  data: u input; SOC output; time input; SOC1 input
function SOC= fcn(u,time,SOC1)
if time <0.006
    SOC= 60 + 60*u/7920;
else
    SOC=SOC1-SOC1*u/7920;
end

== matlab function bus_as_currentsource_charging_discharging_battery_1/Subsystem7/MATLAB Function ==
  data: u input; y output; time input; SOC output; SOC1 input
function [y,SOC]= fcn(u,time,SOC1)
if time <0.006
    SOC= 60 + 60*u/7920;
else
    SOC=SOC1-SOC1*u/7920;
end
y = 5.56e-5.*SOC.^2+0.001788.*SOC+3.491;

== matlab function bus_as_currentsource_charging_discharging_battery_1/Subsystem7/MATLAB Function1 ==
  data: SOC input; y output
function y = fcn(SOC)
p1=2.229e-9;
p2=-5.378e-7;
p3=4.791e-5;
p4=-0.001908;
p5=0.08808;
y=p1*SOC^4+p2*SOC^3+p3*SOC^2+p4*SOC+p5;

== matlab function bus_as_currentsource_charging_discharging_battery_1/Subsystem7/MATLAB Function2 ==
  data: u input; SOC output; time input; SOC1 input
function SOC= fcn(u,time,SOC1)
if time <0.006
    SOC= 60 + 60*u/7920;
else
    SOC=SOC1-SOC1*u/7920;
end

== matlab function bus_as_currentsource_charging_discharging_battery_1/Subsystem8/MATLAB Function ==
  data: u input; y output; time input; SOC output; SOC1 input
function [y,SOC]= fcn(u,time,SOC1)
if time <0.006
    SOC= 60 + 60*u/7920;
else
    SOC=SOC1-SOC1*u/7920;
end
y = 5.56e-5.*SOC.^2+0.001788.*SOC+3.491;

== matlab function bus_as_currentsource_charging_discharging_battery_1/Subsystem1/MATLAB Function1 ==
  data: SOC input; y output
function y = fcn(SOC)
p1=2.229e-9;
p2=-5.378e-7;
p3=4.791e-5;
p4=-0.001908;
p5=0.08808;
y=p1*SOC^4+p2*SOC^3+p3*SOC^2+p4*SOC+p5;

== matlab function bus_as_currentsource_charging_discharging_battery_1/Subsystem8/MATLAB Function1 ==
  data: SOC input; y output
function y = fcn(SOC)
p1=2.229e-9;
p2=-5.378e-7;
p3=4.791e-5;
p4=-0.001908;
p5=0.08808;
y=p1*SOC^4+p2*SOC^3+p3*SOC^2+p4*SOC+p5;

== matlab function bus_as_currentsource_charging_discharging_battery_1/Subsystem8/MATLAB Function2 ==
  data: u input; SOC output; time input; SOC1 input
function SOC= fcn(u,time,SOC1)
if time <0.006
    SOC= 60 + 60*u/7920;
else
    SOC=SOC1-SOC1*u/7920;
end

== matlab function bus_as_currentsource_charging_discharging_battery_1/Subsystem9/MATLAB Function ==
  data: u input; y output; time input; SOC output; SOC1 input
function [y,SOC]= fcn(u,time,SOC1)
if time <0.006
    SOC= 60 + 60*u/7920;
else
    SOC=SOC1-SOC1*u/7920;
end
y = 5.56e-5.*SOC.^2+0.001788.*SOC+3.491;

== matlab function bus_as_currentsource_charging_discharging_battery_1/Subsystem9/MATLAB Function1 ==
  data: SOC input; y output
function y = fcn(SOC)
p1=2.229e-9;
p2=-5.378e-7;
p3=4.791e-5;
p4=-0.001908;
p5=0.08808;
y=p1*SOC^4+p2*SOC^3+p3*SOC^2+p4*SOC+p5;

== matlab function bus_as_currentsource_charging_discharging_battery_1/Subsystem9/MATLAB Function2 ==
  data: u input; SOC output; time input; SOC1 input
function SOC= fcn(u,time,SOC1)
if time <0.006
    SOC= 60 + 60*u/7920;
else
    SOC=SOC1-SOC1*u/7920;
end

== matlab function bus_as_currentsource_charging_discharging_battery_1/Subsystem10/MATLAB Function ==
  data: u input; y output; time input; SOC output; SOC1 input
function [y,SOC]= fcn(u,time,SOC1)
if time <0.006
    SOC= 60 + 60*u/7920;
else
    SOC=SOC1-SOC1*u/7920;
end
y = 5.56e-5.*SOC.^2+0.001788.*SOC+3.491;

== matlab function bus_as_currentsource_charging_discharging_battery_1/Subsystem10/MATLAB Function1 ==
  data: SOC input; y output
function y = fcn(SOC)
p1=2.229e-9;
p2=-5.378e-7;
p3=4.791e-5;
p4=-0.001908;
p5=0.08808;
y=p1*SOC^4+p2*SOC^3+p3*SOC^2+p4*SOC+p5;

== matlab function bus_as_currentsource_charging_discharging_battery_1/Subsystem10/MATLAB Function2 ==
  data: u input; SOC output; time input; SOC1 input
function SOC= fcn(u,time,SOC1)
if time <0.006
    SOC= 60 + 60*u/7920;
else
    SOC=SOC1-SOC1*u/7920;
end

== matlab function bus_as_currentsource_charging_discharging_battery_1/Subsystem1/MATLAB Function2 ==
  data: u input; SOC output; time input; SOC1 input
function SOC= fcn(u,time,SOC1)
if time <0.006
    SOC= 60 + 60*u/7920;
else
    SOC=SOC1-SOC1*u/7920;
end
